simulink subsystem "SimulinkModel"  (R2022b)
settings: Solver=VariableStepAuto  StartTime=0.0  StopTime=10.0  RelTol=1e-3
undefined symbols (not defined in the file): c
settings Model: Creator=is123  LastModifiedBy=is123

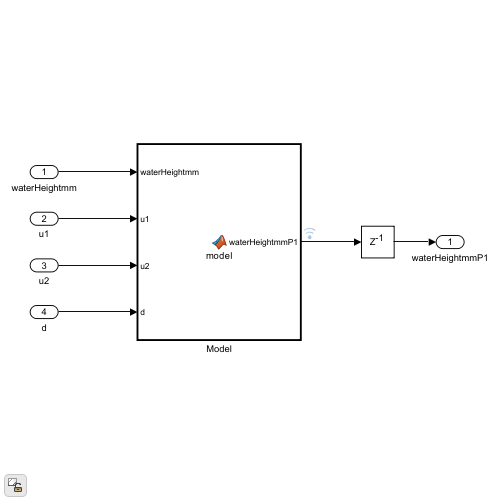
[thumbnail: Simulink's stored preview of the top-level diagram]
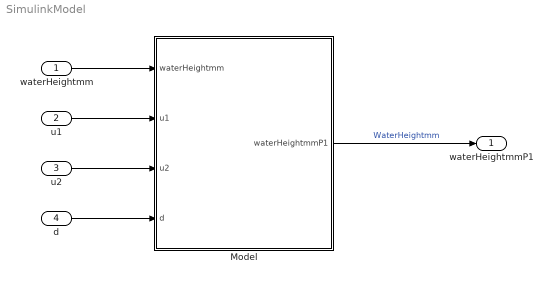
== system SimulinkModel ==
  waterHeightmm : Inport
  u1 : Inport  Port=2
  u2 : Inport  Port=3
  d : Inport  Port=4
  Model : MATLAB Function  TreatAsAtomicUnit=on  SystemSampleTime=3600/c.AccTime
  waterHeightmmP1 : Outport
  wires:
  waterHeightmm/1 -> Model/1(waterHeightmm)
  u1/1 -> Model/2(u1)
  d/1 -> Model/4(d)
  u2/1 -> Model/3(u2)
  Model/1(waterHeightmmP1) -> waterHeightmmP1/1  "WaterHeightmm"

== matlab function SimulinkModel/Model ==
  data: waterHeightmm input; u1 input; u2 input; waterHeightmmP1 output; d input
function waterHeightmmP1 = model(waterHeightmm,u1,u2,d)
%Caling the model function
%Setting the output to zero becuase it is needed
c=scaled_standard_constants;

waterHeightmmP1=zeros(1,1); 
u=[u1;u2];
%calling the model function to get the next volumen
V=waterHeightmm/1e3*c.At;

Vp1=Model(V,u,d);

waterHeightmmP1=Vp1/c.At*1e3; 

end
